simulink model "Circuito_RL_RC_Compensacion_DVG"  (R2017b)
settings: Solver=VariableStepDiscrete  StartTime=0.0  StopTime=1/60*3  MaxStep=1e-4  RelTol=1e-3
libraries: powerlib x9, powerlib_meascontrol x2
settings Model: Creator=DiegoUlises  LastModifiedBy=DiegoUlises

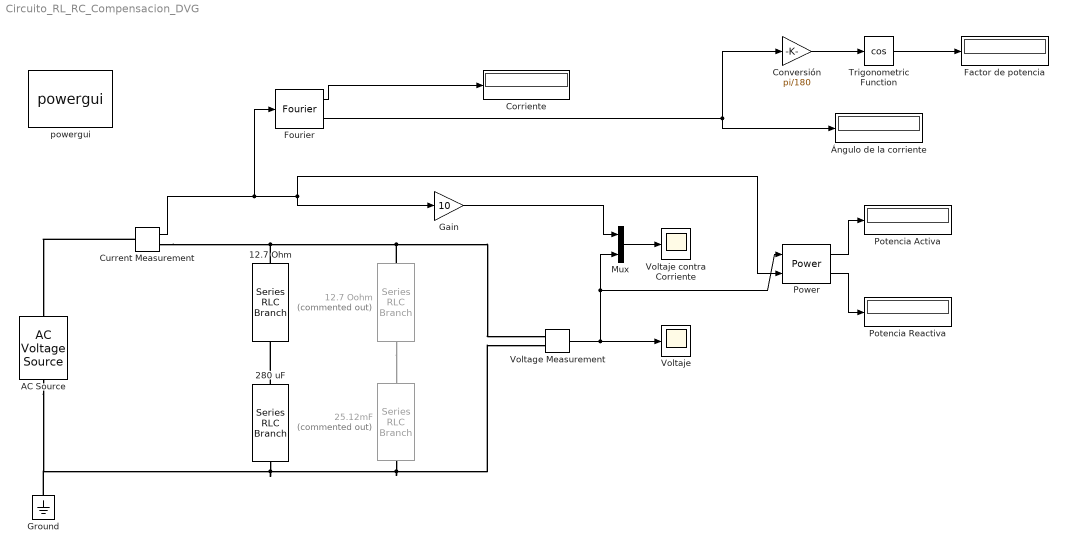
== system Circuito_RL_RC_Compensacion_DVG ==
  12.7 Ohm : powerlib/Elements/Series RLC Branch  LConnTagsString=__new0  RConnTagsString=__new0  BranchType=R  Resistance=12.7  Inductance=50e-3  SetiL0=off  InitialCurrent=0  Capacitance=1e-6  Setx0=off  InitialVoltage=0  Measurements=None
  12.7 Oohm : powerlib/Elements/Series RLC Branch  Commented=on  LConnTagsString=__new0  RConnTagsString=__new0  BranchType=R  Resistance=12.7  Inductance=1e-3  SetiL0=off  InitialCurrent=0  Capacitance=1e-6  Setx0=off  InitialVoltage=0  Measurements=None
  25.12mF : powerlib/Elements/Series RLC Branch  Commented=on  LConnTagsString=__new0  RConnTagsString=__new0  BranchType=L  Resistance=12.7  Inductance=25.12e-3  SetiL0=off  InitialCurrent=0  Capacitance=1e-6  Setx0=off  InitialVoltage=0  Measurements=None
  280 uF : powerlib/Elements/Series RLC Branch  LConnTagsString=__new0  RConnTagsString=__new0  BranchType=C  Resistance=18.7  Inductance=50e-3  SetiL0=off  InitialCurrent=0  Capacitance=280e-6  Setx0=off  InitialVoltage=0  Measurements=None
  AC Source : powerlib/Electrical Sources/AC Voltage Source  Amplitude=311.1269837/1.414213562  Phase=0  Frequency=60  SampleTime=50e-6  Measurements=None  BusType=swing  Pref=10e3  Qref=0  Qmin=-inf  Qmax=+inf
  Conversión : Gain  Gain=pi/180
  "Corriente " : Display
      settings: Decimation=2
  Current Measurement : powerlib/Measurements/Current Measurement  PhasorSimulation=off  OutputType=Complex  PSBequivalent=0
  Factor de potencia : Display
      settings: Decimation=3
  "Fourier " : powerlib_meascontrol/Measurements/Fourier  Freq=60  n=1  InInit=[0, 0]  Ts=50e-6
      settings: SourceProductName=Simscape Power Systems
  "Gain " : Gain  Gain=10
  Ground : powerlib/Elements/Ground  LConnTagsString=a
  Mux : Mux  Inputs=2
  Potencia Activa : Display
      settings: Decimation=2
  Potencia Reactiva : Display
      settings: Decimation=2
  "Power " : powerlib_meascontrol/Measurements/Power  Freq=60  Vinit=[1, 0]  Iinit=[1, 0]  Ts=50e-6
      settings: SourceProductName=Simscape Power Systems
  "Trigonometric Function " : Trigonometry  Operator=cos
  "Voltage Measurement " : powerlib/Measurements/Voltage Measurement  PhasorSimulation=off  OutputType=Complex  PSBequivalent=0
  "Voltaje " : Scope
  Voltaje contra Corriente : Scope
  "powergui " : powerlib/powergui  Priority=1  SimulationMode=Discrete  SampleTime=50e-6  frequency=60  Iterations=50  frequencyindice=60  Pbase=100e6  ErrMax=1e-4  UnitsV=kV  UnitsW=MW  buscounter=0  FunctionMessages=off  echomessages=off  EnableUseOfTLC=off  CurrentSourceSwitches=off  DisableSnubberDevices=off  DisableRonSwitches=off  DisableVfSwitches=off  DisplayEquations=off  SolverType=Tustin/Backward Euler (TBE)  Interpol=off  ExternalGateDelay=off  methode=off  Ts=100  x0status=blocks  SPID=on  SwTol=0  HookPort=off  RestoreLinks=warning  ResistiveCurrentMeasurement=off  Frange=[0:2:500]  Ylog=off  Xlog=on  ShowGrid=off  save=off  variable=ZData  structure=0  ZoomFFT=off  StartTime=0.0  cycles=1  DisplayStyle=1  fundamental=60  FreqAxis=off  MaxFrequency=1000  frequencyindicesteady=1  RmsSteady=1  display=off
  Ángulo de la corriente : Display
      settings: Decimation=2
  wires:
  Current Measurement/1 -> "Fourier "/1, "Power "/2, "Gain "/1
  "Gain "/1 -> Mux/1
  "Voltage Measurement "/1 -> "Voltaje "/1, "Power "/1, Mux/2
  Mux/1 -> Voltaje contra Corriente/1
  "Fourier "/1 -> "Corriente "/1
  "Fourier "/2 -> Conversión/1, Ángulo de la corriente/1
  Conversión/1 -> "Trigonometric Function "/1
  "Trigonometric Function "/1 -> Factor de potencia/1
  "Power "/1 -> Potencia Activa/1
  "Power "/2 -> Potencia Reactiva/1
  connections:
  280 uF/LConn1 -- 12.7 Ohm/RConn1
  12.7 Ohm/LConn1 -- 12.7 Oohm/LConn1 -- "Voltage Measurement "/LConn1 -- Current Measurement/RConn1
  Ground/LConn1 -- AC Source/LConn1 -- 25.12mF/RConn1 -- "Voltage Measurement "/LConn2 -- 280 uF/RConn1
  Current Measurement/LConn1 -- AC Source/RConn1
  12.7 Oohm/RConn1 -- 25.12mF/LConn1
